simulink model "assignment_8_adaptive"  (R2022b)
settings: Solver=VariableStepAuto  StartTime=0.0  StopTime=20  RelTol=1e-3
values from neighbouring files (symbols this model uses):
  A = 1    [assignment_8.m]
  B_hat_initial = get_B_one_dof()*0.7    [assignment_8.m]
  dq0 = [0;0;0]    [assignment_10.m]    (also in assignment_11.m; assignment_12.m; assignment_13.m; assignment_6.m)
  F_hat_initial = get_F_one_dof()*0.7    [assignment_8.m]
  Fc = 1    [assignment_8.m]
  G_hat_initial = get_G_one_dof()*0.7    [assignment_8.m]
  K_D = 10    [assignment_8.m]
  K_theta_inv = inv(K_theta)    [assignment_8.m]
  lambda = 50    [assignment_8.m]
  q0 = [0;0;0]    [assignment_10.m]    (also in assignment_11.m; assignment_12.m; assignment_13.m = [0; pi/2; -pi/2]; assignment_6.m)
  theta = [get_B_one_dof(); get_F_one_dof(); get_G_one_dof]    [assignment_8.m]
undefined symbols (not defined in the file or in its folder): sigbuilder_block
settings Model: Creator=acesi  LastModifiedBy=Manu

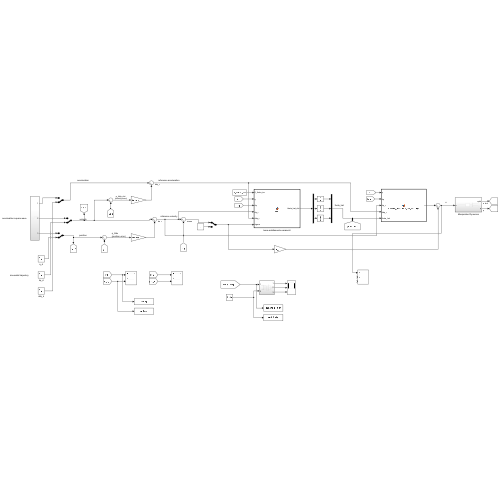
[thumbnail: Simulink's stored preview of the top-level diagram]
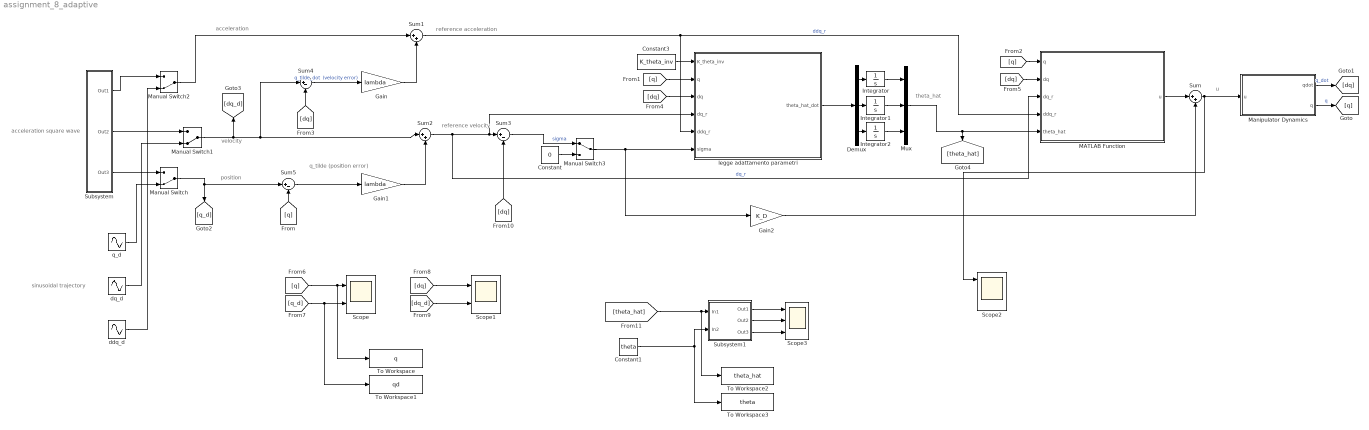
== system assignment_8_adaptive ==
  note: sinusoidal trajectory
  note: acceleration square wave
  note: u
  note: theta_hat
  note: reference acceleration
  note: reference velocity
  note: q_tilde
      | (position error)
  note: acceleration
  note: velocity
  note: position
  Constant : Constant  Value=0
  Constant1 : Constant  Value=theta
  Constant3 : Constant  Value=K_theta_inv
  Demux : Demux  Outputs=3
  Gain : Gain  Gain=lambda
  Gain1 : Gain  Gain=lambda
  Gain2 : Gain  Gain=K_D
  Integrator : Integrator  InitialCondition=B_hat_initial
  Integrator1 : Integrator  InitialCondition=F_hat_initial
  Integrator2 : Integrator  InitialCondition=G_hat_initial
  MATLAB Function : MATLAB Function  TreatAsAtomicUnit=on
  Manipulator Dynamics : Subsystem
  Manual Switch : ManualSwitch  CurrentSetting=0
  Manual Switch1 : ManualSwitch  CurrentSetting=0
  Manual Switch2 : ManualSwitch  CurrentSetting=0
  Manual Switch3 : ManualSwitch
  Mux : Mux  Inputs=3
  Scope : Scope  NumInputPorts=2
  Scope1 : Scope  NumInputPorts=2
  Scope2 : Scope  NumInputPorts=3
  Scope3 : Scope  NumInputPorts=3
  Subsystem : Subsystem
  Subsystem1 : Subsystem
  Sum : Sum  Inputs=|++
  Sum1 : Sum  Inputs=|++
  Sum2 : Sum  Inputs=|++
  Sum3 : Sum  Inputs=|+-
  Sum4 : Sum  Inputs=|+-
  Sum5 : Sum  Inputs=|+-
  To Workspace : ToWorkspace  VariableName=q  SaveFormat=Timeseries  SampleTime=-1
  To Workspace1 : ToWorkspace  VariableName=qd  SaveFormat=Timeseries  SampleTime=-1
  To Workspace2 : ToWorkspace  VariableName=theta_hat  SaveFormat=Timeseries  SampleTime=-1
  To Workspace3 : ToWorkspace  VariableName=theta  SaveFormat=Timeseries  SampleTime=-1
  ddq_d : Sin  Amplitude=-A*Fc*Fc  Frequency=Fc  SampleTime=0
  dq_d : Sin  Amplitude=A*Fc  Frequency=Fc  Phase=pi/2  SampleTime=0
  legge adattamento parametri : MATLAB Function  TreatAsAtomicUnit=on
  q_d : Sin  Amplitude=A  Frequency=Fc  SampleTime=0
  wires:
  Gain/1 -> Sum1/2
  Sum4/1 -> Gain/1  "q_tilde_dot  (velocity error)"
  Sum5/1 -> Gain1/1
  Gain1/1 -> Sum2/2
  Sum2/1 -> Sum3/1, legge adattamento parametri/4(dq_r), MATLAB Function/3(dq_r)  "dq_r"
  Sum1/1 -> legge adattamento parametri/5(ddq_r), MATLAB Function/4(ddq_r)  "ddq_r"
  Constant3/1 -> legge adattamento parametri/1(K_theta_inv)
  legge adattamento parametri/1(theta_hat_dot) -> Demux/1
  Demux/1 -> Integrator/1
  Demux/2 -> Integrator1/1
  Demux/3 -> Integrator2/1
  Integrator/1 -> Mux/1
  Integrator1/1 -> Mux/2
  Integrator2/1 -> Mux/3
  Mux/1 -> MATLAB Function/5(theta_hat), [theta_hat]
  MATLAB Function/1(u) -> Sum/1
  Gain2/1 -> Sum/2
  Sum/1 -> Scope2/1, Manipulator Dynamics/1(u)
  Manipulator Dynamics/2(q) -> [q]  "q"
  Manipulator Dynamics/1(qdot) -> [dq]  "q_dot"
  [q] -> Sum5/2
  [q] -> legge adattamento parametri/2(q)
  [q] -> MATLAB Function/1(q)
  [dq] -> legge adattamento parametri/3(dq)
  [dq] -> MATLAB Function/2(dq)
  [dq] -> Sum4/2
  [q] -> To Workspace/1, Scope/1
  [q_d] -> Scope/2, To Workspace1/1
  [dq_d] -> Scope1/2
  [dq] -> Scope1/1
  Subsystem/3(Out3) -> Manual Switch/1
  Subsystem/2(Out2) -> Manual Switch1/1
  [dq] -> Sum3/2
  Manual Switch/1 -> [q_d], Sum5/1
  q_d/1 -> Manual Switch/2
  Manual Switch1/1 -> [dq_d], Sum4/1, Sum2/1
  dq_d/1 -> Manual Switch1/2
  Subsystem/1(Out1) -> Manual Switch2/1
  Manual Switch2/1 -> Sum1/1
  ddq_d/1 -> Manual Switch2/2
  Constant/1 -> Manual Switch3/2
  Sum3/1 -> Manual Switch3/1  "sigma"
  Manual Switch3/1 -> Gain2/1, legge adattamento parametri/6(sigma)
  [theta_hat] -> To Workspace2/1, Subsystem1/1(In1)
  Constant1/1 -> To Workspace3/1, Subsystem1/2(In2)
  Subsystem1/1(Out1) -> Scope3/1
  Subsystem1/2(Out2) -> Scope3/2
  Subsystem1/3(Out3) -> Scope3/3

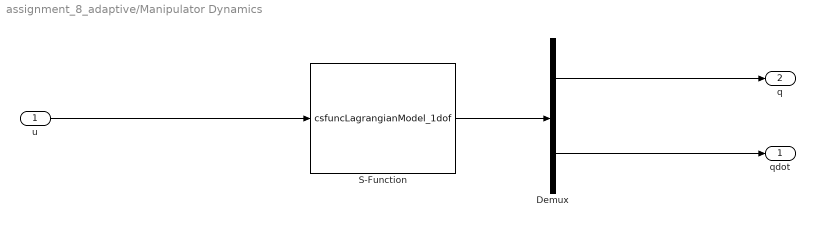
== system assignment_8_adaptive/Manipulator Dynamics ==
  u : Inport
  Demux : Demux  Outputs=2
  S-Function : S-Function  FunctionName=csfuncLagrangianModel_1dof  Parameters=q0 dq0  SFunctionDeploymentMode=off  EnableBusSupport=off
  qdot : Outport
  q : Outport  Port=2
  wires:
  u/1 -> S-Function/1
  S-Function/1 -> Demux/1
  Demux/2 -> qdot/1
  Demux/1 -> q/1

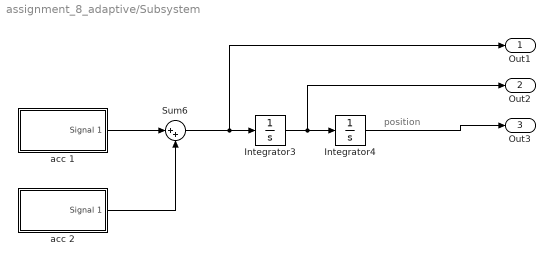
== system assignment_8_adaptive/Subsystem ==
  note: position
  Integrator3 : Integrator
  Integrator4 : Integrator
  Sum6 : Sum  Inputs=|++
  acc 1 : Subsystem  Tag=STV Subsys  LoadFcn=sigbuilder_block('load');  StartFcn=sigbuilder_block('start');  StopFcn=sigbuilder_block('stop');  ClipboardFcn=sigbuilder_block('clipboard');  mask(Sigbuilder block){tuvar=[0:10]}
      mask help: Simulink:masks:SigbuilderBlock_MD
      mask init:
      | if ~strcmp(get_param(bdroot(gcbh),'SimulationStatus'),'stopped') tuvar = sigbuilder_block('maskInit'); end
      settings: CopyFcn=sigbuilder_block('copy');  DeleteFcn=sigbuilder_block('delete');  ModelCloseFcn=sigbuilder_block('modelClose');  PreSaveFcn=sigbuilder_block('preSave');  PauseFcn=sigbuilder_block('pause');  ContinueFcn=sigbuilder_block('continue');  NameChangeFcn=sigbuilder_block('namechange');  OpenFcn=sigbuilder_block('open',[437.6 199.2 550.4 400 ]);  CloseFcn=sigbuilder_block('close');
      mask Display: plot(0, 0, 100, 100,[2, 2, 32, 32, 2], [68, 8, 8, 68, 68],[32, 2], [38, 38], [32, 19, 2],[53, 60, 44], [32, 17, 17, 2],[16, 16, 31, 31]);txt = getActiveGroup(gcbh);text(2, 100, txt,'verticalAlignment', 'top');
  acc 2 : Subsystem  Tag=STV Subsys  LoadFcn=sigbuilder_block('load');  StartFcn=sigbuilder_block('start');  StopFcn=sigbuilder_block('stop');  ClipboardFcn=sigbuilder_block('clipboard');  mask(Sigbuilder block){tuvar=[0:10]}
      mask help: Simulink:masks:SigbuilderBlock_MD
      mask init:
      | if ~strcmp(get_param(bdroot(gcbh),'SimulationStatus'),'stopped') tuvar = sigbuilder_block('maskInit'); end
      settings: CopyFcn=sigbuilder_block('copy');  DeleteFcn=sigbuilder_block('delete');  ModelCloseFcn=sigbuilder_block('modelClose');  PreSaveFcn=sigbuilder_block('preSave');  PauseFcn=sigbuilder_block('pause');  ContinueFcn=sigbuilder_block('continue');  NameChangeFcn=sigbuilder_block('namechange');  OpenFcn=sigbuilder_block('open',[403.5 84.75 550.5 363.75 ]);  CloseFcn=sigbuilder_block('close');
      mask Display: plot(0, 0, 100, 100,[2, 2, 32, 32, 2], [68, 8, 8, 68, 68],[32, 2], [38, 38], [32, 19, 2],[53, 60, 44], [32, 17, 17, 2],[16, 16, 31, 31]);txt = getActiveGroup(gcbh);text(2, 100, txt,'verticalAlignment', 'top');
  Out1 : Outport
  Out2 : Outport  Port=2
  Out3 : Outport  Port=3
  wires:
  Sum6/1 -> Out1/1, Integrator3/1
  acc 2/1(Signal 1) -> Sum6/2
  Integrator4/1 -> Out3/1
  Integrator3/1 -> Out2/1, Integrator4/1
  acc 1/1(Signal 1) -> Sum6/1

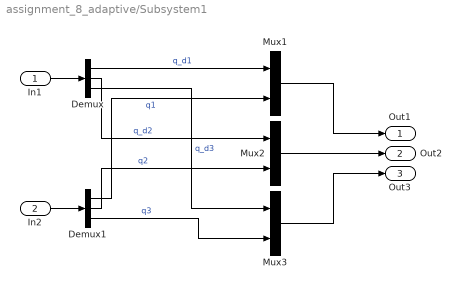
== system assignment_8_adaptive/Subsystem1 ==
  In1 : Inport
  In2 : Inport  Port=2
  Demux : Demux  Outputs=3
  Demux1 : Demux  Outputs=3
  Mux1 : Mux  Inputs=2
  Mux2 : Mux  Inputs=2
  Mux3 : Mux  Inputs=2
  Out1 : Outport
  Out2 : Outport  Port=2
  Out3 : Outport  Port=3
  wires:
  Demux/1 -> Mux1/1  "q_d1"
  Demux/3 -> Mux3/1  "q_d3"
  Demux/2 -> Mux2/1  "q_d2"
  Demux1/1 -> Mux1/2  "q1"
  Mux2/1 -> Out2/1
  Demux1/3 -> Mux3/2  "q3"
  Demux1/2 -> Mux2/2  "q2"
  Mux3/1 -> Out3/1
  Mux1/1 -> Out1/1
  In2/1 -> Demux1/1
  In1/1 -> Demux/1

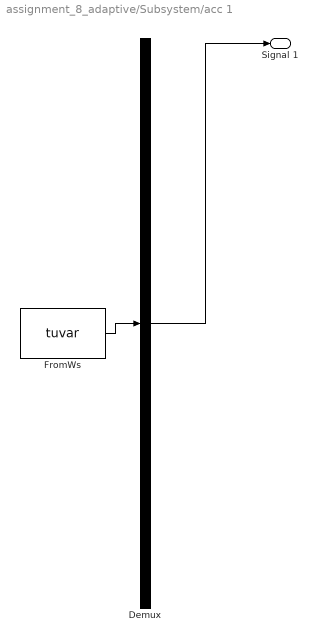
== system assignment_8_adaptive/Subsystem/acc 1 ==
  Demux : Demux  Tag=STV Demux  Outputs=1
      settings: DisplayOption=none
  FromWs : FromWorkspace  Tag=STV FromWs  VariableName=tuvar
      SigBuilderData=|
      | common.afterFinalStr = 'Extrapolate'
      | common.sampleTime = 0
      | dataSet.timeRange = [0 10]
      | dataSet.name = 'Group 1'
      | sbobj.Groups.Name = 'Group 1'
      | sbobj.Groups.Signals.Name = 'Signal 1'
      | sbobj.Groups.Signals.XData = [0 1 1 3 3 10]
      | sbobj.Groups.Signals.YData = [0 0 1 1 0 0]
  Signal 1 : Outport  Tag=STV Outport
  wires:
  Demux/1 -> Signal 1/1
  FromWs/1 -> Demux/1

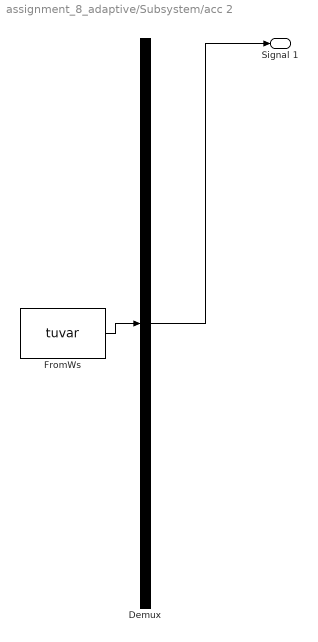
== system assignment_8_adaptive/Subsystem/acc 2 ==
  Demux : Demux  Tag=STV Demux  Outputs=1
      settings: DisplayOption=none
  FromWs : FromWorkspace  Tag=STV FromWs  VariableName=tuvar
      SigBuilderData=|
      | common.afterFinalStr = 'Extrapolate'
      | common.sampleTime = 0
      | dataSet.timeRange = [0 10]
      | dataSet.name = 'Group 1'
      | sbobj.Groups.Name = 'Group 1'
      | sbobj.Groups.Signals.Name = 'Signal 1'
      | sbobj.Groups.Signals.XData = [0 6 6 9 9 10]
      | sbobj.Groups.Signals.YData = [0 0 -1 -1 0 0]
  Signal 1 : Outport  Tag=STV Outport
  wires:
  Demux/1 -> Signal 1/1
  FromWs/1 -> Demux/1

== matlab function assignment_8_adaptive/MATLAB Function ==
  data: q input; dq input; u output; dq_r input; ddq_r input; theta_hat input
function u = inverse_dynamics_ctrl_strategy(q, dq, dq_r, ddq_r, theta_hat)
    % NB: knowing theta is like knowing B, C, F, G
    % Y * theta_hat è un'azione di controllo simile a quella dello schema 
    % a dinamica inversa (dove ci sono B ed n (n = C+F+G))
    % quindi facendo Y*theta_hat facciamo una approssimazione degli effetti
    % non lineari e il disaccoppiamento tra i giunti
    % però in maniera approssimativa perchè non abbiamo theta, ma theta_hat
    Y = get_Y(q, dq_r, ddq_r);
    u = Y * theta_hat;
end

== matlab function assignment_8_adaptive/legge adattamento parametri ==
  data: K_theta_inv input; q input; theta_hat_dot output; dq input; dq_r input; ddq_r input; sigma input
function theta_hat_dot = fcn(K_theta_inv, q, dq, dq_r, ddq_r, sigma)
    Y = get_Y(q, dq_r, ddq_r);
    theta_hat_dot = K_theta_inv * Y' * sigma;
end
